simulink model "Practica3_simulink"  (R2024a)
settings: Solver=VariableStepAuto  StartTime=0.0  StopTime=15  RelTol=1e-3
settings Model: Creator=danid
settings RTWCC: GPUComputeCapability=3.5

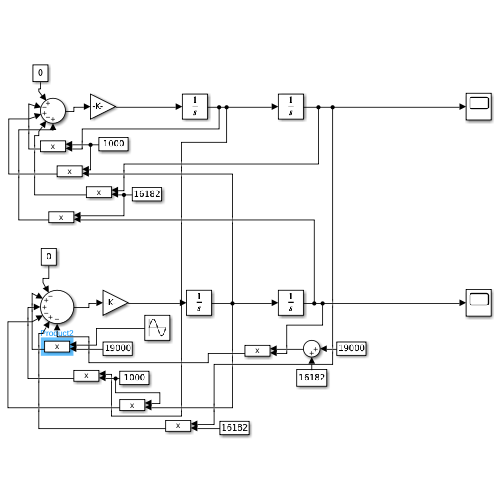
[thumbnail: Simulink's stored preview of the top-level diagram]
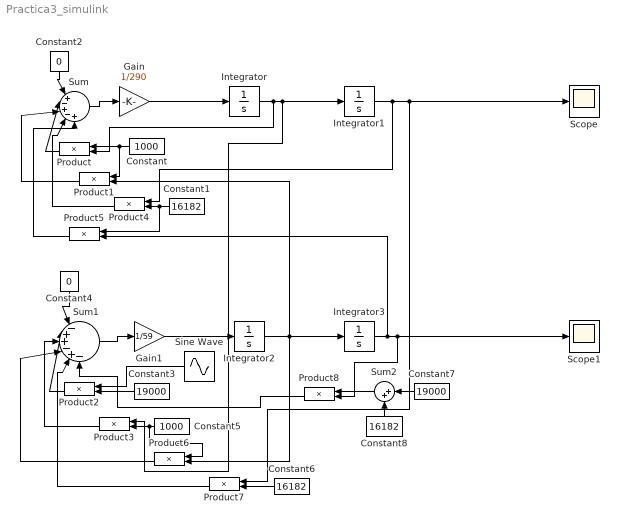
== system Practica3_simulink ==
  Constant : Constant  Value=1000
  Constant1 : Constant  Value=16182
  Constant2 : Constant  Value=0
  Constant3 : Constant  Value=19000
  Constant4 : Constant  Value=0
  Constant5 : Constant  Value=1000
  Constant6 : Constant  Value=16182
  Constant7 : Constant  Value=19000
  Constant8 : Constant  Value=16182
  Gain : Gain  Gain=1/290
  Gain1 : Gain  Gain=1/59
  Integrator{,1..3} (4 alike) : Integrator
  Product{,1..8} (9 alike) : Product
  Scope : Scope
  Scope1 : Scope
  Sine Wave : Sin  Amplitude=.05  Frequency=.5*pi  SampleTime=0
  Sum : Sum  Inputs=|+-+-+
  Sum1 : Sum  Inputs=|-++-+-
  Sum2 : Sum  Inputs=|++
  wires:
  Sum/1 -> Gain/1
  Gain/1 -> Integrator/1
  Integrator/1 -> Product/2, Product3/1, Integrator1/1
  Constant/1 -> Product1/1, Product/1
  Product/1 -> Sum/2
  Gain1/1 -> Integrator2/1
  Product2/1 -> Sum1/2
  Sum1/1 -> Gain1/1
  Integrator2/1 -> Product1/2, Integrator3/1, Product6/2
  Product1/1 -> Sum/3
  Constant1/1 -> Product5/1, Product4/2
  Product4/1 -> Sum/4
  Product5/1 -> Sum/5
  Constant2/1 -> Sum/1
  Constant4/1 -> Sum1/1
  Constant5/1 -> Product6/1, Product3/2
  Constant3/1 -> Product2/2
  Product3/1 -> Sum1/3
  Product6/1 -> Sum1/4
  Constant6/1 -> Product7/2
  Product7/1 -> Sum1/5
  Sum2/1 -> Product8/1
  Constant8/1 -> Sum2/2
  Constant7/1 -> Sum2/1
  Product8/1 -> Sum1/6
  Integrator1/1 -> Product4/1, Product7/1, Scope/1
  Integrator3/1 -> Product5/2, Product8/2, Scope1/1
  Sine Wave/1 -> Product2/1
